simulink model "H89"  (Simulink 7.3)
settings: Solver=ode45  StartTime=0.0  StopTime=2  RelTol=1e-3
libraries: simulink x1
settings Model: Creator=Sainquake  LastModifiedBy=Sainquake

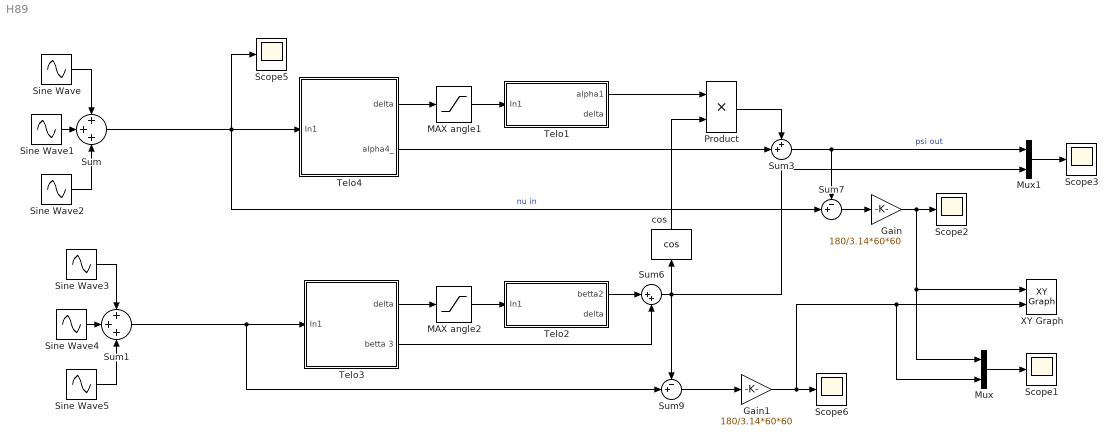
== system H89 ==
  Gain : Gain  Gain=180/3.14*60*60  ParameterDataType=fixdt(1, 16)  ParameterScaling=2^0  OutDataType=fixdt(1, 16)  OutScaling=2^0
  Gain1 : Gain  Gain=180/3.14*60*60  ParameterDataType=fixdt(1, 16)  ParameterScaling=2^0  OutDataType=fixdt(1, 16)  OutScaling=2^0
  MAX angle1 : Saturate  UpperLimit=3/180*3.14  LowerLimit=-3/180*3.14
  MAX angle2 : Saturate  UpperLimit=3/180*3.14  LowerLimit=-3/180*3.14
  Mux : Mux  Inputs=2
  Mux1 : Mux  Inputs=2
  Product : Product  OutDataType=fixdt(1, 16)  OutScaling=2^0  RndMeth=Zero
  Scope{1..3,5..6} (5 alike) : Scope
      Scope1 settings: YMin=-10000  YMax=120000  MaxDataPoints=50000
      Scope2 settings: YMin=25000  YMax=65000  SaveName=ScopeData2  MaxDataPoints=50000
      Scope3 settings: YMin=0.72  YMax=0.835  MaxDataPoints=50000
      Scope5 settings: YMin=-0.375  YMax=0.025  SaveName=ScopeData5  MaxDataPoints=50000
      Scope6 settings: YMin=25000  YMax=65000  SaveName=ScopeData6  MaxDataPoints=50000
  Sine Wave : Sin  Amplitude=0.8  Bias=0  Frequency=1  Phase=0  Samples=10  SampleTime=0  Offset=0
  Sine Wave1 : Sin  Amplitude=1/60  Bias=0  Frequency=2*pi*14  Phase=0  Samples=10  SampleTime=0  Offset=0
  Sine Wave2 : Sin  Amplitude=1/60  Bias=0  Frequency=2*pi*4  Phase=0  Samples=10  SampleTime=0  Offset=0
  Sine Wave3 : Sin  Amplitude=0.8  Bias=0  Frequency=1  Phase=pi/2  Samples=10  SampleTime=0  Offset=0
  Sine Wave4 : Sin  Amplitude=1/60  Bias=0  Frequency=2*pi*14  Phase=pi/2  Samples=10  SampleTime=0  Offset=0
  Sine Wave5 : Sin  Amplitude=1/60  Bias=0  Frequency=2*pi*4  Phase=pi/2  Samples=10  SampleTime=0  Offset=0
  Sum : Sum  Inputs=+++  OutDataType=fixdt(1, 16)  OutScaling=2^0
  Sum1 : Sum  Inputs=+++  OutDataType=fixdt(1, 16)  OutScaling=2^0
  Sum3 : Sum  Inputs=++|  OutDataType=fixdt(1, 16)  OutScaling=2^0
  Sum6 : Sum  Inputs=|++  OutDataType=fixdt(1, 16)  OutScaling=2^0
  Sum7 : Sum  Inputs=-+|  OutDataType=fixdt(1, 16)  OutScaling=2^0
  Sum9 : Sum  Inputs=-+|  OutDataType=fixdt(1, 16)  OutScaling=2^0
  Telo1 : Subsystem
  Telo2 : Subsystem
  Telo3 : Subsystem
  Telo4 : Subsystem
  XY Graph : simulink/Sinks/XY Graph  SystemSampleTime=-1  xmin=-3*1280  xmax=3*1280  ymin=-3*960  ymax=3*960  st=-1
  cos : Trigonometry  Operator=cos
  wires:
  Product/1 -> Sum3/1
  Sum3/1 -> Sum7/1, Mux1/1  "psi out"
  Sum6/1 -> Sum9/1, cos/1, Mux1/2
  Sum7/1 -> Gain/1
  Gain/1 -> Scope2/1, XY Graph/1, Mux/1
  cos/1 -> Product/2
  Sum/1 -> Scope5/1, Sum7/2, Telo4/1(In1)  "nu in"
  MAX angle1/1 -> Telo1/1(In1)
  Sine Wave/1 -> Sum/1
  Sine Wave2/1 -> Sum/3
  Sine Wave1/1 -> Sum/2
  Gain1/1 -> Scope6/1, XY Graph/2, Mux/2
  MAX angle2/1 -> Telo2/1(In1)
  Telo4/1(delta) -> MAX angle1/1
  Telo4/2(alpha4_) -> Sum3/2
  Telo3/1(delta) -> MAX angle2/1
  Telo3/2(betta 3) -> Sum6/2
  Telo1/1(alpha1) -> Product/1
  Telo2/1(betta2) -> Sum6/1
  Sum9/1 -> Gain1/1
  Mux/1 -> Scope1/1
  Mux1/1 -> Scope3/1
  Sum1/1 -> Telo3/1(In1), Sum9/2
  Sine Wave3/1 -> Sum1/1
  Sine Wave5/1 -> Sum1/3
  Sine Wave4/1 -> Sum1/2

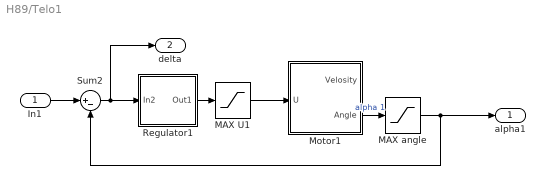
== system H89/Telo1 ==
  In1 : Inport  OutDataType=fixdt(1, 16)  OutScaling=2^0
  MAX U1 : Saturate  UpperLimit=12  LowerLimit=-12
  MAX angle : Saturate  UpperLimit=4/180*3.14  LowerLimit=-4/180*3.14
  Motor1 : Subsystem  TreatAsAtomicUnit=on
  Regulator1 : Subsystem
  Sum2 : Sum  Inputs=|+-  OutDataType=fixdt(1, 16)  OutScaling=2^0
  alpha1 : Outport  OutDataType=fixdt(1, 16)  OutScaling=2^0
  delta : Outport  Port=2  OutDataType=fixdt(1, 16)  OutScaling=2^0
  wires:
  Motor1/2(Angle) -> MAX angle/1  "alpha 1"
  Sum2/1 -> delta/1, Regulator1/1(In2)
  MAX U1/1 -> Motor1/1(U)
  MAX angle/1 -> Sum2/2, alpha1/1
  In1/1 -> Sum2/1
  Regulator1/1(Out1) -> MAX U1/1

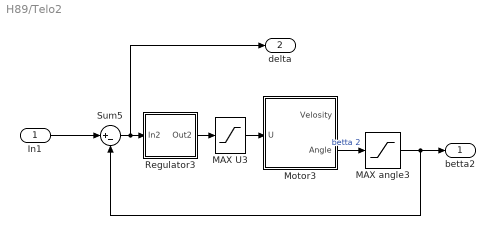
== system H89/Telo2 ==
  In1 : Inport  OutDataType=fixdt(1, 16)  OutScaling=2^0
  MAX U3 : Saturate  UpperLimit=12  LowerLimit=-12
  MAX angle3 : Saturate  UpperLimit=4/180*3.14  LowerLimit=-4/180*3.14
  Motor3 : Subsystem  TreatAsAtomicUnit=on
  Regulator3 : Subsystem
  Sum5 : Sum  Inputs=|+-  OutDataType=fixdt(1, 16)  OutScaling=2^0
  betta2 : Outport  OutDataType=fixdt(1, 16)  OutScaling=2^0
  delta : Outport  Port=2  OutDataType=fixdt(1, 16)  OutScaling=2^0
  wires:
  Sum5/1 -> delta/1, Regulator3/1(In2)
  MAX U3/1 -> Motor3/1(U)
  MAX angle3/1 -> Sum5/2, betta2/1
  Motor3/2(Angle) -> MAX angle3/1  "betta 2"
  In1/1 -> Sum5/1
  Regulator3/1(Out2) -> MAX U3/1

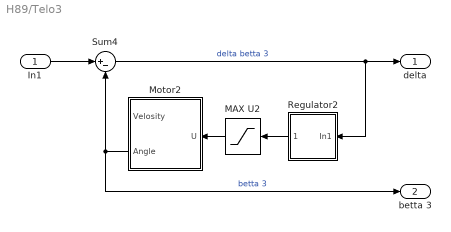
== system H89/Telo3 ==
  In1 : Inport  OutDataType=fixdt(1, 16)  OutScaling=2^0
  MAX U2 : Saturate  UpperLimit=27  LowerLimit=-27
  Motor2 : Subsystem  TreatAsAtomicUnit=on
  Regulator2 : Subsystem
  Sum4 : Sum  Inputs=|+-  OutDataType=fixdt(1, 16)  OutScaling=2^0
  delta : Outport  OutDataType=fixdt(1, 16)  OutScaling=2^0
  betta 3 : Outport  Port=2  OutDataType=fixdt(1, 16)  OutScaling=2^0
  wires:
  Sum4/1 -> delta/1, Regulator2/1(In1)  "delta betta 3"
  Motor2/2(Angle) -> Sum4/2, betta 3/1  "betta 3"
  MAX U2/1 -> Motor2/1(U)
  In1/1 -> Sum4/1
  Regulator2/1(Out1) -> MAX U2/1

== system H89/Telo4 ==
  In1 : Inport  OutDataType=fixdt(1, 16)  OutScaling=2^0
  MAX U : Saturate  UpperLimit=27  LowerLimit=-27
  Motor : Subsystem  TreatAsAtomicUnit=on
  Regulator : Subsystem
  Sum1 : Sum  Inputs=|+-  OutDataType=fixdt(1, 16)  OutScaling=2^0
  delta : Outport  OutDataType=fixdt(1, 16)  OutScaling=2^0
  alpha4_ : Outport  Port=2  OutDataType=fixdt(1, 16)  OutScaling=2^0
  wires:
  Sum1/1 -> delta/1, MAX U/1  "delta alpha 4"
  Motor/2(Angle) -> Sum1/2, alpha4_/1  "alpha 4"
  MAX U/1 -> Motor/1(U)
  In1/1 -> Sum1/1

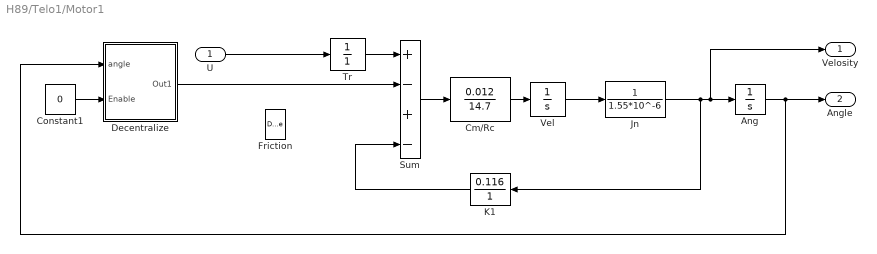
== system H89/Telo1/Motor1 ==
  U : Inport  OutDataType=fixdt(1, 16)  OutScaling=2^0
  Ang : Integrator
  Cm/Rc : TransferFcn  Numerator=[0.012]  Denominator=14.7
  Constant1 : Constant  Value=0  OutDataType=fixdt(1, 16)  OutScaling=2^0
  Decentralize : Subsystem  TreatAsAtomicUnit=on
  Friction : DeadZone  LowerValue=-1.4  UpperValue=1.4  SaturateOnIntegerOverflow=on
  Jn : TransferFcn  Denominator=1.55*10^-6
  K1 : TransferFcn  Numerator=0.116  Denominator=[ 1]
  Sum : Sum  Inputs=+-+-
  Tr : TransferFcn  Numerator=1  Denominator=[ 1 ]
  Vel : Integrator
  Velosity : Outport  OutDataType=fixdt(1, 16)  OutScaling=2^0
  Angle : Outport  Port=2  OutDataType=fixdt(1, 16)  OutScaling=2^0
  wires:
  Sum/1 -> Cm/Rc/1
  Ang/1 -> Decentralize/1(angle), Angle/1
  K1/1 -> Sum/4
  Tr/1 -> Sum/1
  Decentralize/1(Out1) -> Sum/2
  Constant1/1 -> Decentralize/2(Enable)
  Jn/1 -> K1/1, Ang/1, Velosity/1
  Cm/Rc/1 -> Vel/1
  Vel/1 -> Jn/1
  U/1 -> Tr/1

== system H89/Telo1/Regulator1 ==
  In2 : Inport  OutDataType=fixdt(1, 16)  OutScaling=2^0
  Gain1 : Gain  Gain=41  ParameterDataType=fixdt(1, 16)  ParameterScaling=2^0  OutDataType=fixdt(1, 16)  OutScaling=2^0
  Gain2 : Gain  Gain=8100  ParameterDataType=fixdt(1, 16)  ParameterScaling=2^0  OutDataType=fixdt(1, 16)  OutScaling=2^0
  Transfer Fcn : TransferFcn  Numerator=[0.01 1]  Denominator=[0.0001 1]
  Transfer Fcn1 : TransferFcn  Numerator=[0.003 1]  Denominator=[0.00005 1]
  Out1 : Outport  OutDataType=fixdt(1, 16)  OutScaling=2^0
  wires:
  Gain1/1 -> Transfer Fcn/1
  ? -> Gain1/1
  Transfer Fcn/1 -> ?
  Gain2/1 -> Transfer Fcn1/1
  In2/1 -> Gain2/1
  Transfer Fcn1/1 -> Out1/1

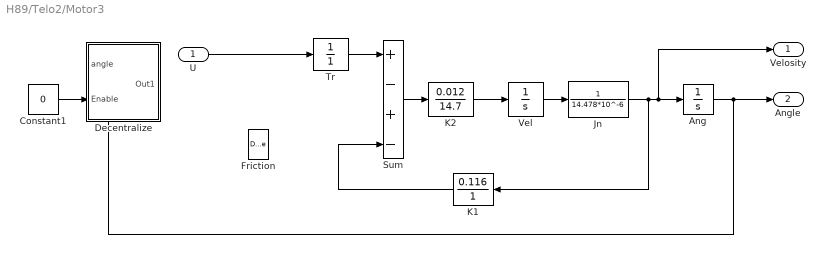
== system H89/Telo2/Motor3 ==
  U : Inport  OutDataType=fixdt(1, 16)  OutScaling=2^0
  Ang : Integrator
  Constant1 : Constant  Value=0  OutDataType=fixdt(1, 16)  OutScaling=2^0
  Decentralize : Subsystem  TreatAsAtomicUnit=on
  Friction : DeadZone  LowerValue=-1.4  UpperValue=1.4  SaturateOnIntegerOverflow=on
  Jn : TransferFcn  Denominator=14.478*10^-6
  K1 : TransferFcn  Numerator=0.116  Denominator=[ 1]
  K2 : TransferFcn  Numerator=0.012  Denominator=14.7
  Sum : Sum  Inputs=+-+-
  Tr : TransferFcn  Numerator=1  Denominator=[ 1 ]
  Vel : Integrator
  Velosity : Outport  OutDataType=fixdt(1, 16)  OutScaling=2^0
  Angle : Outport  Port=2  OutDataType=fixdt(1, 16)  OutScaling=2^0
  wires:
  Sum/1 -> K2/1
  K2/1 -> Vel/1
  Ang/1 -> Decentralize/1(angle), Angle/1
  K1/1 -> Sum/4
  Tr/1 -> Sum/1
  U/1 -> Tr/1
  Constant1/1 -> Decentralize/2(Enable)
  Vel/1 -> Jn/1
  Jn/1 -> K1/1, Ang/1, Velosity/1

== system H89/Telo2/Regulator3 ==
  In2 : Inport  OutDataType=fixdt(1, 16)  OutScaling=2^0
  Gain2 : Gain  Gain=8100  ParameterDataType=fixdt(1, 16)  ParameterScaling=2^0  OutDataType=fixdt(1, 16)  OutScaling=2^0
  Transfer Fcn1 : TransferFcn  Numerator=[0.003 1]  Denominator=[0.00005 1]
  Out2 : Outport  OutDataType=fixdt(1, 16)  OutScaling=2^0
  wires:
  Gain2/1 -> Transfer Fcn1/1
  In2/1 -> Gain2/1
  Transfer Fcn1/1 -> Out2/1

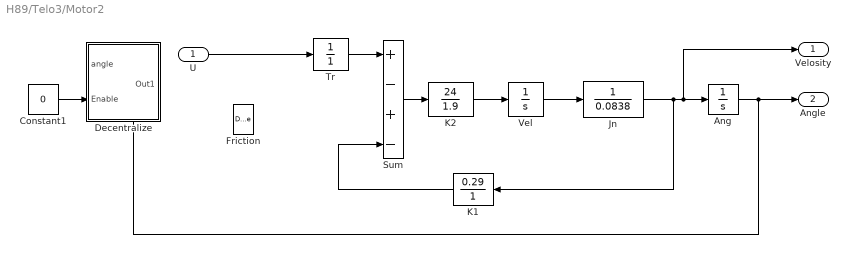
== system H89/Telo3/Motor2 ==
  U : Inport  OutDataType=fixdt(1, 16)  OutScaling=2^0
  Ang : Integrator
  Constant1 : Constant  Value=0  OutDataType=fixdt(1, 16)  OutScaling=2^0
  Decentralize : Subsystem  TreatAsAtomicUnit=on
  Friction : DeadZone  LowerValue=-1.4  UpperValue=1.4  SaturateOnIntegerOverflow=on
  Jn : TransferFcn  Denominator=0.0838
  K1 : TransferFcn  Numerator=0.29  Denominator=[ 1]
  K2 : TransferFcn  Numerator=24  Denominator=1.9
  Sum : Sum  Inputs=+-+-
  Tr : TransferFcn  Numerator=1  Denominator=[ 1 ]
  Vel : Integrator
  Velosity : Outport  OutDataType=fixdt(1, 16)  OutScaling=2^0
  Angle : Outport  Port=2  OutDataType=fixdt(1, 16)  OutScaling=2^0
  wires:
  Sum/1 -> K2/1
  K2/1 -> Vel/1
  Ang/1 -> Decentralize/1(angle), Angle/1
  K1/1 -> Sum/4
  Tr/1 -> Sum/1
  U/1 -> Tr/1
  Constant1/1 -> Decentralize/2(Enable)
  Vel/1 -> Jn/1
  Jn/1 -> K1/1, Ang/1, Velosity/1

== system H89/Telo3/Regulator2 ==
  In1 : Inport  OutDataType=fixdt(1, 16)  OutScaling=2^0
  Gain : Gain  Gain=60  ParameterDataType=fixdt(1, 16)  ParameterScaling=2^0  OutDataType=fixdt(1, 16)  OutScaling=2^0
  Transfer Fcn : TransferFcn  Numerator=[15/60 1]  Denominator=[0.001 1]
  Out1 : Outport  OutDataType=fixdt(1, 16)  OutScaling=2^0
  wires:
  Gain/1 -> Transfer Fcn/1
  In1/1 -> Gain/1
  Transfer Fcn/1 -> Out1/1

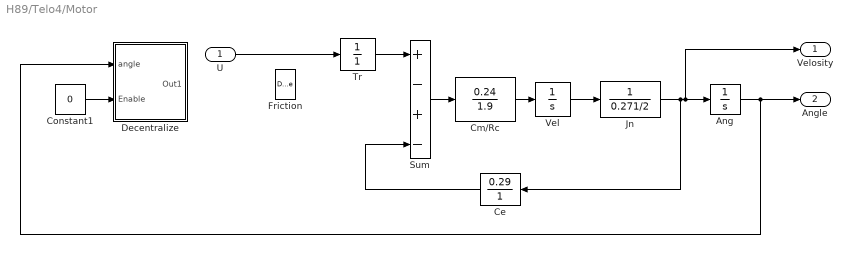
== system H89/Telo4/Motor ==
  U : Inport  OutDataType=fixdt(1, 16)  OutScaling=2^0
  Ang : Integrator
  Ce : TransferFcn  Numerator=[0.29]  Denominator=[ 1]
  Cm/Rc : TransferFcn  Numerator=[0.24]  Denominator=1.9
  Constant1 : Constant  Value=0  OutDataType=fixdt(1, 16)  OutScaling=2^0
  Decentralize : Subsystem  TreatAsAtomicUnit=on
  Friction : DeadZone  LowerValue=-1.4  UpperValue=1.4  SaturateOnIntegerOverflow=on
  Jn : TransferFcn  Denominator=0.271/2
  Sum : Sum  Inputs=+-+-
  Tr : TransferFcn  Denominator=[ 1 ]
  Vel : Integrator
  Velosity : Outport  OutDataType=fixdt(1, 16)  OutScaling=2^0
  Angle : Outport  Port=2  OutDataType=fixdt(1, 16)  OutScaling=2^0
  wires:
  Sum/1 -> Cm/Rc/1
  Cm/Rc/1 -> Vel/1
  Ang/1 -> Decentralize/1(angle), Angle/1
  Ce/1 -> Sum/4
  Tr/1 -> Sum/1
  Constant1/1 -> Decentralize/2(Enable)
  Vel/1 -> Jn/1
  Jn/1 -> Ce/1, Ang/1, Velosity/1
  U/1 -> Tr/1

== system H89/Telo4/Regulator ==
  In1 : Inport  OutDataType=fixdt(1, 16)  OutScaling=2^0
  Gain : Gain  Gain=60  ParameterDataType=fixdt(1, 16)  ParameterScaling=2^0  OutDataType=fixdt(1, 16)  OutScaling=2^0
  Transfer Fcn : TransferFcn  Numerator=[15/60 1]  Denominator=[0.001 1]
  Out1 : Outport  OutDataType=fixdt(1, 16)  OutScaling=2^0
  wires:
  In1/1 -> Gain/1
  Gain/1 -> Transfer Fcn/1
  Transfer Fcn/1 -> Out1/1

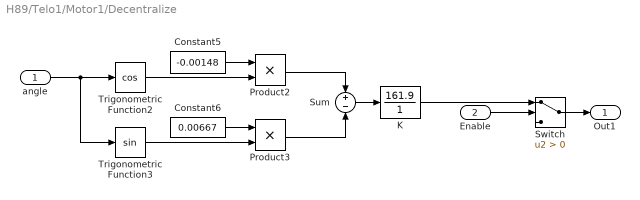
== system H89/Telo1/Motor1/Decentralize ==
  angle : Inport  OutDataType=fixdt(1, 16)  OutScaling=2^0
  Enable : Inport  Port=2  OutDataType=fixdt(1, 16)  OutScaling=2^0
  Constant5 : Constant  Value=-0.00148
  Constant6 : Constant  Value=0.00667
  K : TransferFcn  Numerator=[161.9]  Denominator=[ 1 ]
  Product2 : Product  RndMeth=Zero
  Product3 : Product  RndMeth=Zero
  Sum : Sum  Inputs=+|-  OutDataType=fixdt(1, 16)  OutScaling=2^0
  Switch : Switch  Criteria=u2 > Threshold  OutDataType=fixdt(1, 16)  OutScaling=2^0
  Trigonometric Function2 : Trigonometry  Operator=cos
  Trigonometric Function3 : Trigonometry
  Out1 : Outport  OutDataType=fixdt(1, 16)  OutScaling=2^0
  wires:
  Constant5/1 -> Product2/1
  Trigonometric Function2/1 -> Product2/2
  Constant6/1 -> Product3/1
  Trigonometric Function3/1 -> Product3/2
  Product3/1 -> Sum/2
  Product2/1 -> Sum/1
  Sum/1 -> K/1
  K/1 -> Switch/1
  angle/1 -> Trigonometric Function2/1, Trigonometric Function3/1
  Enable/1 -> Switch/2
  Switch/1 -> Out1/1

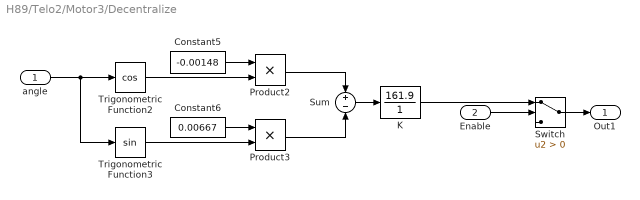
== system H89/Telo2/Motor3/Decentralize ==
  angle : Inport  OutDataType=fixdt(1, 16)  OutScaling=2^0
  Enable : Inport  Port=2  OutDataType=fixdt(1, 16)  OutScaling=2^0
  Constant5 : Constant  Value=-0.00148
  Constant6 : Constant  Value=0.00667
  K : TransferFcn  Numerator=[161.9]  Denominator=[ 1 ]
  Product2 : Product  RndMeth=Zero
  Product3 : Product  RndMeth=Zero
  Sum : Sum  Inputs=+|-  OutDataType=fixdt(1, 16)  OutScaling=2^0
  Switch : Switch  Criteria=u2 > Threshold  OutDataType=fixdt(1, 16)  OutScaling=2^0
  Trigonometric Function2 : Trigonometry  Operator=cos
  Trigonometric Function3 : Trigonometry
  Out1 : Outport  OutDataType=fixdt(1, 16)  OutScaling=2^0
  wires:
  Constant5/1 -> Product2/1
  Trigonometric Function2/1 -> Product2/2
  Constant6/1 -> Product3/1
  Trigonometric Function3/1 -> Product3/2
  Product3/1 -> Sum/2
  Product2/1 -> Sum/1
  Sum/1 -> K/1
  K/1 -> Switch/1
  angle/1 -> Trigonometric Function2/1, Trigonometric Function3/1
  Enable/1 -> Switch/2
  Switch/1 -> Out1/1

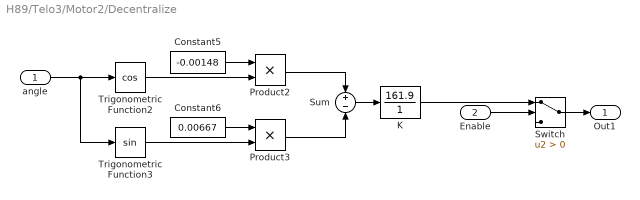
== system H89/Telo3/Motor2/Decentralize ==
  angle : Inport  OutDataType=fixdt(1, 16)  OutScaling=2^0
  Enable : Inport  Port=2  OutDataType=fixdt(1, 16)  OutScaling=2^0
  Constant5 : Constant  Value=-0.00148
  Constant6 : Constant  Value=0.00667
  K : TransferFcn  Numerator=[161.9]  Denominator=[ 1 ]
  Product2 : Product  RndMeth=Zero
  Product3 : Product  RndMeth=Zero
  Sum : Sum  Inputs=+|-  OutDataType=fixdt(1, 16)  OutScaling=2^0
  Switch : Switch  Criteria=u2 > Threshold  OutDataType=fixdt(1, 16)  OutScaling=2^0
  Trigonometric Function2 : Trigonometry  Operator=cos
  Trigonometric Function3 : Trigonometry
  Out1 : Outport  OutDataType=fixdt(1, 16)  OutScaling=2^0
  wires:
  Constant5/1 -> Product2/1
  Trigonometric Function2/1 -> Product2/2
  Constant6/1 -> Product3/1
  Trigonometric Function3/1 -> Product3/2
  Product3/1 -> Sum/2
  Product2/1 -> Sum/1
  Sum/1 -> K/1
  K/1 -> Switch/1
  angle/1 -> Trigonometric Function2/1, Trigonometric Function3/1
  Enable/1 -> Switch/2
  Switch/1 -> Out1/1

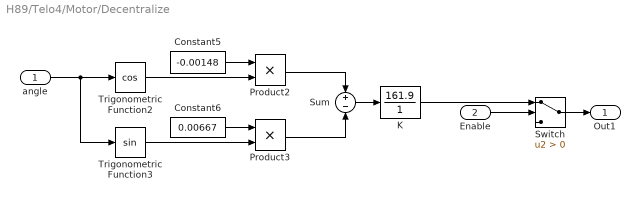
== system H89/Telo4/Motor/Decentralize ==
  angle : Inport  OutDataType=fixdt(1, 16)  OutScaling=2^0
  Enable : Inport  Port=2  OutDataType=fixdt(1, 16)  OutScaling=2^0
  Constant5 : Constant  Value=-0.00148
  Constant6 : Constant  Value=0.00667
  K : TransferFcn  Numerator=[161.9]  Denominator=[ 1 ]
  Product2 : Product  RndMeth=Zero
  Product3 : Product  RndMeth=Zero
  Sum : Sum  Inputs=+|-  OutDataType=fixdt(1, 16)  OutScaling=2^0
  Switch : Switch  Criteria=u2 > Threshold  OutDataType=fixdt(1, 16)  OutScaling=2^0
  Trigonometric Function2 : Trigonometry  Operator=cos
  Trigonometric Function3 : Trigonometry
  Out1 : Outport  OutDataType=fixdt(1, 16)  OutScaling=2^0
  wires:
  Constant5/1 -> Product2/1
  Trigonometric Function2/1 -> Product2/2
  Constant6/1 -> Product3/1
  Trigonometric Function3/1 -> Product3/2
  Product3/1 -> Sum/2
  Product2/1 -> Sum/1
  Sum/1 -> K/1
  K/1 -> Switch/1
  angle/1 -> Trigonometric Function2/1, Trigonometric Function3/1
  Enable/1 -> Switch/2
  Switch/1 -> Out1/1
